simulink model "scCO2_exact"  (R2024a)
settings: Solver=ode4  StartTime=0.0  StopTime=9000  FixedStep=0.1  RelTol=1e-3
libraries: simulink x1
settings Model: Creator=Vijai Venkatesh  LastModifiedBy=Vijai Venkatesh

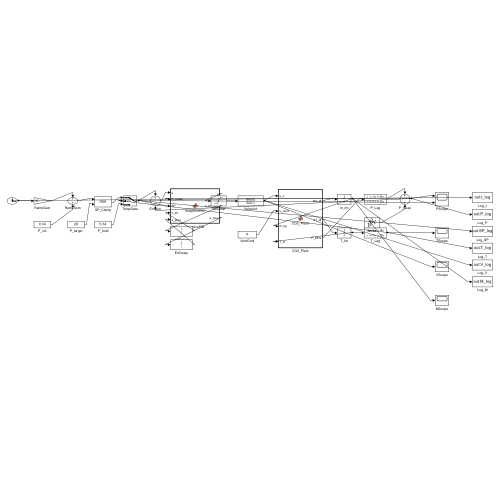
[thumbnail: Simulink's stored preview of the top-level diagram]
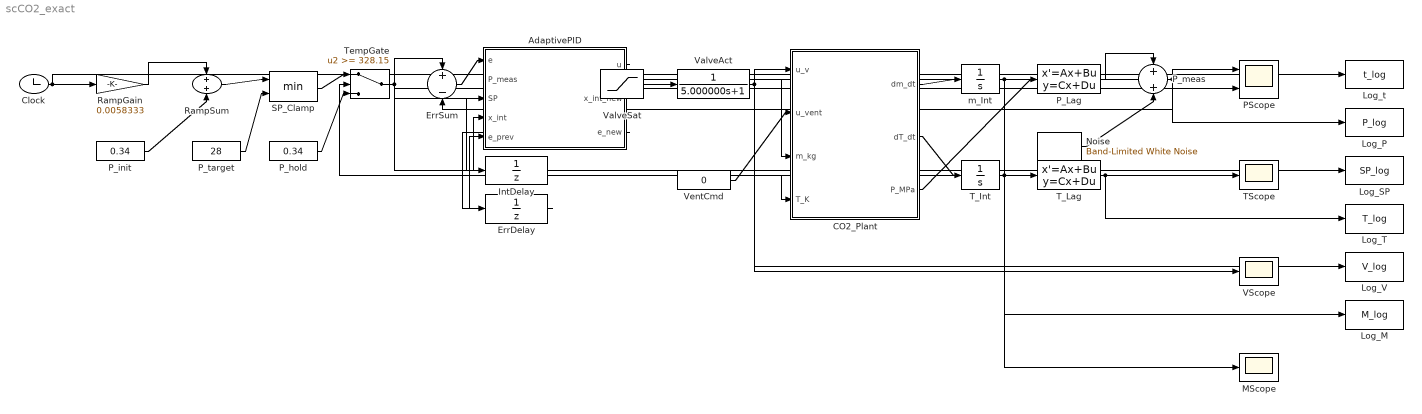
== system scCO2_exact ==
  AdaptivePID : MATLAB Function  TreatAsAtomicUnit=on
  CO2_Plant : MATLAB Function  TreatAsAtomicUnit=on
  Clock : Clock
  ErrDelay : UnitDelay  SampleTime=0.1  HasFrameUpgradeWarning=on
  ErrSum : Sum  Inputs=+-
  IntDelay : UnitDelay  SampleTime=0.1  HasFrameUpgradeWarning=on
  Log_M : ToWorkspace  VariableName=M_log  SampleTime=0.1
  Log_P : ToWorkspace  VariableName=P_log  SampleTime=0.1
  Log_SP : ToWorkspace  VariableName=SP_log  SampleTime=0.1
  Log_T : ToWorkspace  VariableName=T_log  SampleTime=0.1
  Log_V : ToWorkspace  VariableName=V_log  SampleTime=0.1
  Log_t : ToWorkspace  VariableName=t_log  SampleTime=0.1
  MScope : Scope
  Noise : simulink/Sources/Band-Limited White Noise  Cov=2.5e-6  Ts=0.1  seed=12345
  PScope : Scope  NumInputPorts=2
  P_Lag : StateSpace  A=-20  B=20  D=0  InitialCondition=0.34
  P_hold : Constant  Value=0.34
  P_init : Constant  Value=0.34
  P_meas : Sum
  P_target : Constant  Value=28
  RampGain : Gain  Gain=0.0058333
  RampSum : Sum
  SP_Clamp : MinMax  Inputs=2
  TScope : Scope
  T_Int : Integrator  InitialCondition=298.15
  T_Lag : StateSpace  A=-0.033333  B=0.033333  D=0  InitialCondition=298.15
  TempGate : Switch  Threshold=328.15  SaturateOnIntegerOverflow=off  InputSameDT=off
  VScope : Scope
  ValveAct : TransferFcn  Denominator=[5.000000 1]
  ValveSat : Saturate  UpperLimit=100  LowerLimit=0
  VentCmd : Constant  Value=0
  m_Int : Integrator  InitialCondition=0.0060791
  wires:
  Clock/1 -> RampGain/1, Log_t/1
  RampGain/1 -> RampSum/1
  P_init/1 -> RampSum/2
  RampSum/1 -> SP_Clamp/1
  P_target/1 -> SP_Clamp/2
  SP_Clamp/1 -> TempGate/1
  T_Lag/1 -> TempGate/2, TScope/1, Log_T/1
  P_hold/1 -> TempGate/3
  TempGate/1 -> ErrSum/1, AdaptivePID/3(SP), PScope/2, Log_SP/1
  P_meas/1 -> ErrSum/2, AdaptivePID/2(P_meas), PScope/1, Log_P/1
  ErrSum/1 -> AdaptivePID/1(e)
  IntDelay/1 -> AdaptivePID/4(x_int)
  ErrDelay/1 -> AdaptivePID/5(e_prev)
  AdaptivePID/1(u) -> ValveSat/1
  AdaptivePID/2(x_int_new) -> IntDelay/1
  AdaptivePID/3(e_new) -> ErrDelay/1
  ValveSat/1 -> ValveAct/1
  ValveAct/1 -> CO2_Plant/1(u_v), VScope/1, Log_V/1
  VentCmd/1 -> CO2_Plant/2(u_vent)
  m_Int/1 -> CO2_Plant/3(m_kg), MScope/1, Log_M/1
  T_Int/1 -> CO2_Plant/4(T_K), T_Lag/1
  CO2_Plant/1(dm_dt) -> m_Int/1
  CO2_Plant/2(dT_dt) -> T_Int/1
  CO2_Plant/3(P_MPa) -> P_Lag/1
  P_Lag/1 -> P_meas/1
  Noise/1 -> P_meas/2

== matlab function scCO2_exact/CO2_Plant ==
  data: u_v input; dm_dt output; u_vent input; m_kg input; T_K input; dT_dt output; P_MPa output
function [dm_dt, dT_dt, P_MPa] = CO2_Plant(u_v, u_vent, m_kg, T_K)
% PR-EOS (van der Waals mixing) + mass/energy balance
% Pure gas (CO2, N2, or Ar)  |  INKBIRD heater  |  TiO2 nanofluid
R_M=8.314;
% Component critical properties and kappa
Tc=[304.13,126.192,150.86]; Pc=[7.377e6,3.3958e6,4.898e6]; kp=[0.7080,0.4316,0.3746];
% Mole fractions (embedded at build time)
y=[1.000000,0.000000,0.000000];
% Binary interaction params (CO2-N2, CO2-Ar, N2-Ar)
kij_12=0.028000; kij_13=0.124000; kij_23=0.000000;
% Hardware + mixture constants (embedded at build time)
V_ves=1.000000e-03; K_valve=1.202000e-07; K_vent=2.404000e-07;
UA_wall=3.000; T_env_K=298.150; P_boost=2.800000e+07; rho_boost=984.6117;
Cv_sp=900.00; Cp_sp=1100.00; M_mix=0.044010; b_mix=2.66666890e-05;
UA_inkbird=50.000; T_inkbird_K=333.150; M_therm=250.000; TiO2_phi=0.000000;
a0=[3.962808e-01,1.482128e-01,1.468567e-01];
% State guards
m=max(m_kg,1e-2); T=max(min(T_K,1200),200);
% PR-EOS a_mix(T) — van der Waals mixing (unrolled for codegen)
alph=(1+kp.*(1-sqrt(T./Tc))).^2;
a_T=a0.*alph;
a_mix=y(1)^2*a_T(1)+y(2)^2*a_T(2)+y(3)^2*a_T(3)...
     +2*y(1)*y(2)*sqrt(a_T(1)*a_T(2))*(1-kij_12)...
     +2*y(1)*y(3)*sqrt(a_T(1)*a_T(3))*(1-kij_13)...
     +2*y(2)*y(3)*sqrt(a_T(2)*a_T(3))*(1-kij_23);
% PR-EOS: P from (rho, T) — molar volume from mass density
rho_mol=(m/V_ves)/M_mix;
Vm=1/rho_mol;
Vm_s=max(Vm,b_mix*1.001);
P_Pa=R_M*T/(Vm_s-b_mix)-a_mix/(Vm_s*(Vm_s+b_mix)+b_mix*(Vm_s-b_mix));
P_Pa=max(P_Pa,1e4); P_MPa=P_Pa/1e6;
% Effective density with TiO2 volume fraction
rho=m/V_ves;
rho_eff=(1-TiO2_phi)*rho+TiO2_phi*4230;
% Valve flow in
dP_in=max(P_boost-P_Pa,0);
mdot_in=K_valve*(u_v/100)*sqrt(2*rho_boost*dP_in);
% Vent flow out
dP_out=max(P_Pa-1.013e5,0);
mdot_out=K_vent*(u_vent/100)*sqrt(2*max(rho_eff,0.1)*dP_out);
% Mass balance
dm_dt=mdot_in-mdot_out;
% Energy balance: inlet enthalpy + compression work + wall loss + INKBIRD
h_diff=Cp_sp*(T_env_K-T);
Q_wall=UA_wall*(T_env_K-T);
Q_inkbird=UA_inkbird*max(T_inkbird_K-T,0);
comp_W=dm_dt*P_Pa/max(rho_eff,0.1);
denom=max(m*Cv_sp+M_therm,1e-2);
dT_raw=(mdot_in*h_diff+comp_W+Q_wall+Q_inkbird)/denom;
dT_dt=max(min(dT_raw,200),-200);
end

== matlab function scCO2_exact/AdaptivePID ==
  data: e input; u output; P_meas input; SP input; x_int input; e_prev input; x_int_new output; e_new output
function [u, x_int_new, e_new] = AdaptivePID(e, P_meas, SP, x_int, e_prev)
% Stateless adaptive gain-scheduled PID — state held by Unit Delay blocks.
% No persistent variables => no sample-time restrictions.
Ts=0.1; N=20; P_TARGET=28.0; Kb=0.1;
% Two-regime gain schedule (2500 psi = 17.2 MPa crossover):
%   0-17.2 MPa: gains RISE  (high compressibility, needs more flow)
%  17.2-28 MPa: gains FALL  (dense fluid, hair-trigger response)
P_bp  = [0,   5,   10,  17.2, 20,  24,  27,  28 ];
Kp_bp = [50,  58,  65,  60,   45,  32,  22,  18 ];
Ki_bp = [6,   7,   8,   7,    5,   4,   3,   3  ];
Kd_bp = [2.5, 2.5, 2.0, 1.5,  1.0, 0.8, 0.5, 0.5];
in_hold = (SP >= P_TARGET - 0.02);
if in_hold
    Kp=35.0; Ki=12.0; Kd=0.5;
else
    P_c = max(0, min(P_meas, P_bp(end)));
    Kp = interp1(P_bp, Kp_bp, P_c, 'linear');
    Ki = interp1(P_bp, Ki_bp, P_c, 'linear');
    Kd = interp1(P_bp, Kd_bp, P_c, 'linear');
end
de = (e - e_prev) / Ts;
de_f = de * N / (1 + N*Ts);
u_raw = Kp*e + Ki*x_int + Kd*de_f;
u = max(min(u_raw, 100), 0);
x_int_new = x_int + Ts*e + Ts*Kb*(u - u_raw);
e_new = e;
end
